simulink model "simex5"  (R2023b)
settings: Solver=VariableStepAuto  StartTime=0.0  StopTime=20  RelTol=1e-3
undefined symbols (not defined in the file or in its folder): DiscIntNeverNeededParam
libraries: simulink x7
settings Model: PacingRate=0.220000  Creator=Vinar  LastModifiedBy=Vinar
settings OptimizationCC: ReuseModelBlockBuffer=off

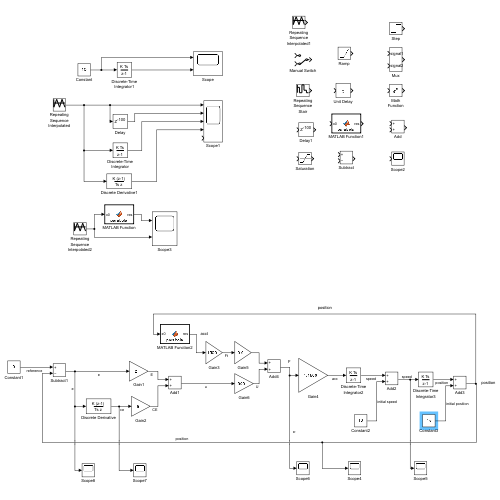
[thumbnail: Simulink's stored preview of the top-level diagram]
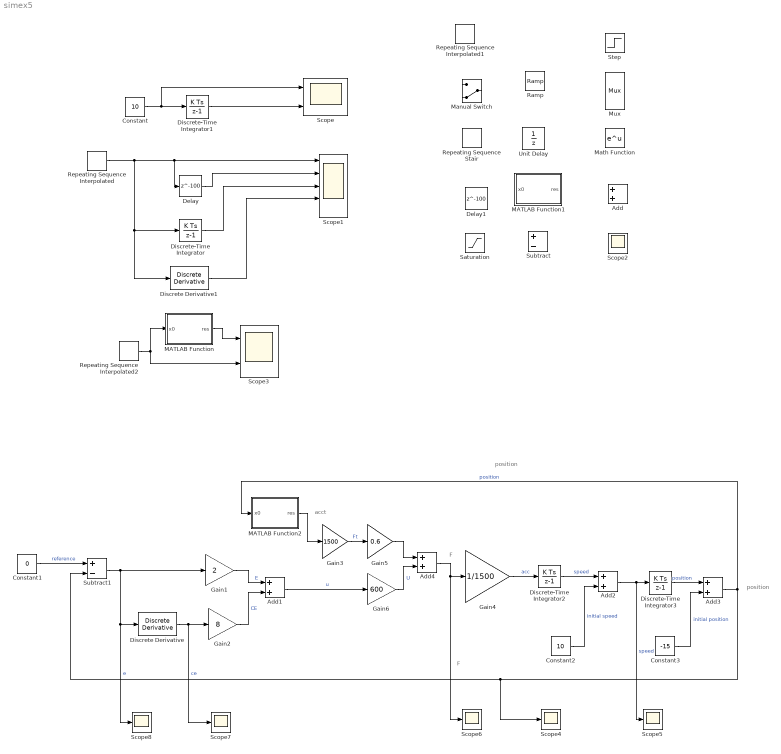
== system simex5 ==
  note: F
  note: position
  note: position
  note: acct
  note: F
  Add{,1..4} (5 alike) : Sum
  Constant : Constant  Value=10  SampleTime=1
  Constant1 : Constant  Value=0
  Constant2 : Constant  Value=10
  Constant3 : Constant  Value=-15
  Delay : Delay  DelayLength=100  InitialCondition=-100  SampleTime=0.1
  Delay1 : Delay  DelayLength=100  InitialCondition=-100  SampleTime=0.1
  Discrete Derivative : simulink/Discrete/Discrete Derivative  gainval=1.0  ICPrevScaledInput=150  OutMin=[]  OutMax=[]  OutDataType=fixdt(1, 16)  OutScaling=2^-10  DoSatur=off
  Discrete Derivative1 : simulink/Discrete/Discrete Derivative  gainval=1.0  ICPrevScaledInput=-1000  OutMin=[]  OutMax=[]  OutDataType=fixdt(1, 16)  OutScaling=2^-10  DoSatur=off
  Discrete-Time Integrator : DiscreteIntegrator  SampleTime=0.1  ICPrevOutput=DiscIntNeverNeededParam  ICPrevScaledInput=DiscIntNeverNeededParam
  Discrete-Time Integrator1 : DiscreteIntegrator  ICPrevOutput=DiscIntNeverNeededParam  ICPrevScaledInput=DiscIntNeverNeededParam
  Discrete-Time Integrator2 : DiscreteIntegrator  SampleTime=0.1  ICPrevOutput=DiscIntNeverNeededParam  ICPrevScaledInput=DiscIntNeverNeededParam
  Discrete-Time Integrator3 : DiscreteIntegrator  SampleTime=0.1  ICPrevOutput=DiscIntNeverNeededParam  ICPrevScaledInput=DiscIntNeverNeededParam
  Gain1 : Gain  Gain=2
  Gain2 : Gain  Gain=8
  Gain3 : Gain  Gain=1500
  Gain4 : Gain  Gain=1/1500
  Gain5 : Gain  Gain=0.6
  Gain6 : Gain  Gain=600
  MATLAB Function : MATLAB Function  TreatAsAtomicUnit=on
  MATLAB Function1 : MATLAB Function  TreatAsAtomicUnit=on
  MATLAB Function2 : MATLAB Function  TreatAsAtomicUnit=on
  Manual Switch : ManualSwitch  CurrentSetting=0
  Math Function : Math
  Mux : Mux  Inputs=2
      settings: DisplayOption=signals
  Ramp : simulink/Sources/Ramp  slope=1  start=0  InitialOutput=0
  Repeating Sequence Interpolated : simulink/Sources/Repeating Sequence Interpolated  OutValues=[-100 100 -100 100 -100].'  TimeValues=[0 50 100 150 200].'  LookUpMeth=Interpolation-Use End Values  tsamp=0.1  OutMin=[]  OutMax=[]  OutDataTypeStr=double  OutputDataTypeScalingMode=double  OutDataType=fixdt(0,8)  OutScaling=2^-10
  Repeating Sequence Interpolated1 : simulink/Sources/Repeating Sequence Interpolated  OutValues=[-100 100 -100 100 -100].'  TimeValues=[0 50 100 150 200].'  LookUpMeth=Interpolation-Use End Values  tsamp=0.1  OutMin=[]  OutMax=[]  OutDataTypeStr=double  OutputDataTypeScalingMode=double  OutDataType=fixdt(0,8)  OutScaling=2^-10
  Repeating Sequence Interpolated2 : simulink/Sources/Repeating Sequence Interpolated  OutValues=[-10 10 -10 10 -10].'  TimeValues=[0 50 100 150 200].'  LookUpMeth=Interpolation-Use End Values  tsamp=0.1  OutMin=[]  OutMax=[]  OutDataTypeStr=double  OutputDataTypeScalingMode=double  OutDataType=fixdt(0,8)  OutScaling=2^-10
  Repeating Sequence Stair : simulink/Sources/Repeating Sequence Stair  OutValues=[3 1 4 2 1].'  tsamp=-1  OutMin=[]  OutMax=[]  OutDataTypeStr=double  OutputDataTypeScalingMode=double  OutDataType=fixdt(0,8)  ConRadixGroup=Best Precision: Vector-wise  OutScaling=2^-12
  Saturation : Saturate
  Scope : Scope  NumInputPorts=2
  Scope1 : Scope  NumInputPorts=5
  Scope{2,4..8} (6 alike) : Scope
  Scope3 : Scope  NumInputPorts=2
  Step : Step  SampleTime=0
  Subtract : Sum  Inputs=+-
  Subtract1 : Sum  Inputs=+-
  Unit Delay : UnitDelay  SampleTime=-1  HasFrameUpgradeWarning=on
  wires:
  Delay/1 -> Scope1/2
  Repeating Sequence Interpolated/1 -> Scope1/1, Delay/1, Discrete Derivative1/1, Discrete-Time Integrator/1
  Discrete-Time Integrator/1 -> Scope1/3
  Constant/1 -> Scope/1, Discrete-Time Integrator1/1
  Discrete-Time Integrator1/1 -> Scope/2
  Discrete Derivative1/1 -> Scope1/4
  Constant1/1 -> Subtract1/1  "reference"
  Subtract1/1 -> Scope8/1, Discrete Derivative/1, Gain1/1  "e"
  Discrete Derivative/1 -> Gain2/1, Scope7/1  "ce"
  Gain2/1 -> Add1/2  "CE"
  Add1/1 -> Gain6/1  "u"
  Gain4/1 -> Discrete-Time Integrator2/1  "acc"
  Add4/1 -> Scope6/1, Gain4/1
  Discrete-Time Integrator2/1 -> Add2/1  "speed"
  Add2/1 -> Scope5/1, Discrete-Time Integrator3/1  "speed"
  Discrete-Time Integrator3/1 -> Add3/1  "position"
  Add3/1 -> MATLAB Function2/1(x0), Subtract1/2, Scope4/1  "position"
  Constant2/1 -> Add2/2  "initial speed"
  Constant3/1 -> Add3/2  "initial position"
  MATLAB Function/1(res) -> Scope3/1
  Repeating Sequence Interpolated2/1 -> Scope3/2, MATLAB Function/1(x0)
  Gain6/1 -> Add4/2  "U"
  MATLAB Function2/1(res) -> Gain3/1
  Gain3/1 -> Gain5/1  "Ft"
  Gain5/1 -> Add4/1
  Gain1/1 -> Add1/1  "E"

== matlab function simex5/MATLAB Function ==
  data: x0 input; res output
function res=parabola(x0)
gc=9.81;
ap=2;
t1=-gc*2*ap*x0/(1+4*ap^2*x0^2);
res=sqrt(1+4*ap^2*x0^2)*t1;

== matlab function simex5/MATLAB Function2 ==
  data: x0 input; res output
function res=parabola(x0)
gc=9.81;
ap=2;
t1=-gc*2*ap*x0/(1+4*ap^2*x0^2);
if x0>=0
 res=-sqrt(1+4*ap^2*x0^2)*abs(t1);
else
 res=sqrt(1+4*ap^2*x0^2)*abs(t1);
end
end

== matlab function simex5/MATLAB Function1 ==
  data: x0 input; res output
function res=parabola(x0)
gc=9.81;
ap=2;
t1=-gc/(2*ap*x0+1/(2*ap*x0));
res=sqrt(1+4*ap^2*x0^2)*t1;
